simulink model "RightTrajectoryAgent"  (Simulink 6.5)
settings: Solver=ode45  SolverMode=SingleTasking  StartTime=0.0  StopTime=10.0  RelTol=1e-3  AbsTol=1e-6
settings Model: Creator=The MathWorks Inc.  LastModifiedBy=suarezjl  ExtModeTrigMode=oneshot  ExtModeArmWhenConnect=off  ExtModeAutoUpdateStatusClock=off
settings DataIOCC: LimitDataPoints=off  SignalLoggingName=logsOut
settings OptimizationCC: BooleanDataType=off  InlineInvariantSignals=on
settings DebuggingCC: CheckExecutionContextPreStartOutputMsg=on  CheckExecutionContextRuntimeOutputMsg=on  SolverPrmCheckMsg=none  MultiTaskDSMMsg=warning  MultiTaskCondExecSysMsg=none  IntegerOverflowMsg=none  StrictBusMsg=None
settings HardwareCC: TargetUnknown=on
settings ModelReferenceCC: UpdateModelReferenceTargets=IfOutOfDate
settings RTWCC: IncludeERTFirstTime=on

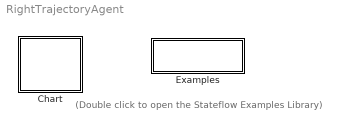
== system RightTrajectoryAgent ==
  note: (Double click to open the
      | Stateflow Examples Library)
  Chart : Stateflow chart
  Examples : Subsystem
      settings: OpenFcn=sf('Private','sf_examples')
      mask Display: disp('Examples')

== system RightTrajectoryAgent/Examples ==

== stateflow chart Chart ==
  state InitializeFunctions
    Hungerforce\RightReachDemo\RightTrajectoryAgent\LoadHomePosition.Initialize()
    Hungerforce\RightReachDemo\RightTrajectoryAgent\PlayCurrentTraj.Initialize()
    Hungerforce\RightReachDemo\RightTrajectoryAgent\LoadHomePosition.Write2VS()
  state CopyCurrentLocation
    Hungerforce\RightReachDemo\RightTrajectoryAgent\CopyGoalPosition.CopyRowVector()
    Hungerforce\RightReachDemo\RightTrajectoryAgent\CopyCurrentPosition.CopyCurrentVector()
  state GenerateCurrentTrajectory
    Hungerforce\RightReachDemo\RightTrajectoryAgent\GenerateCurrentTraj.GenerateTrajectory()
  state PlayCurrentTrajectory
    Hungerforce\RightReachDemo\RightTrajectoryAgent\PlayCurrentTraj.OutputTrajectory()
    Hungerforce\RightReachDemo\RightTrajectoryAgent\StateMachine.Wait(10000)
  state CopyHomeLocation
    Hungerforce\RightReachDemo\RightTrajectoryAgent\CopyHomePosition.CopyRowVector()
    Hungerforce\RightReachDemo\RightTrajectoryAgent\CopyCurrentPosition.CopyCurrentVector()
  state PlayHomeTrajectory
    Hungerforce\RightReachDemo\RightTrajectoryAgent\PlayCurrentTraj.OutputTrajectory()
  state GenerateHomeTrajectory
    Hungerforce\RightReachDemo\RightTrajectoryAgent\GenerateCurrentTraj.GenerateTrajectory()
  state Check that object is seen
    Hungerforce\RightReachDemo\RightTrajectoryAgent\GenerateCurrentTraj.CheckForObject()
  (default) -> InitializeFunctions : Start
  InitializeFunctions -> Check that object is seen : Always
  CopyCurrentLocation -> GenerateCurrentTrajectory : Always
  GenerateCurrentTrajectory -> PlayCurrentTrajectory : Always
  PlayHomeTrajectory -> CopyCurrentLocation : Signal="Next"
  PlayCurrentTrajectory -> CopyHomeLocation : Always
  GenerateHomeTrajectory -> PlayHomeTrajectory : Signal="Next"
  CopyHomeLocation -> GenerateHomeTrajectory : Always
  Check that object is seen -> CopyCurrentLocation : Signal ="Next"
